simulink model "QuarterModelSimulink"  (R2017a)
settings: Solver=VariableStepAuto  StartTime=0.0  StopTime=20  RelTol=1e-3
values from neighbouring files (symbols this model uses):
  c_s = 2 * zeta * sqrt(k_u*m_s)    [simulink_main.m]
  k_s = k_u * 5    (= 34897655.371)    [simulink_main.m]
  k_u = k_u_eng * Pa_over_psi    (= 6979531.0742)    [simulink_main.m]
  m_s = 1109 / 4    (= 277.25)    [simulink_main.m]
  m_u = m_u_extra + m_rubber + m_air    [simulink_main.m]
settings Model: Creator=alexkost  LastModifiedBy=alexkost

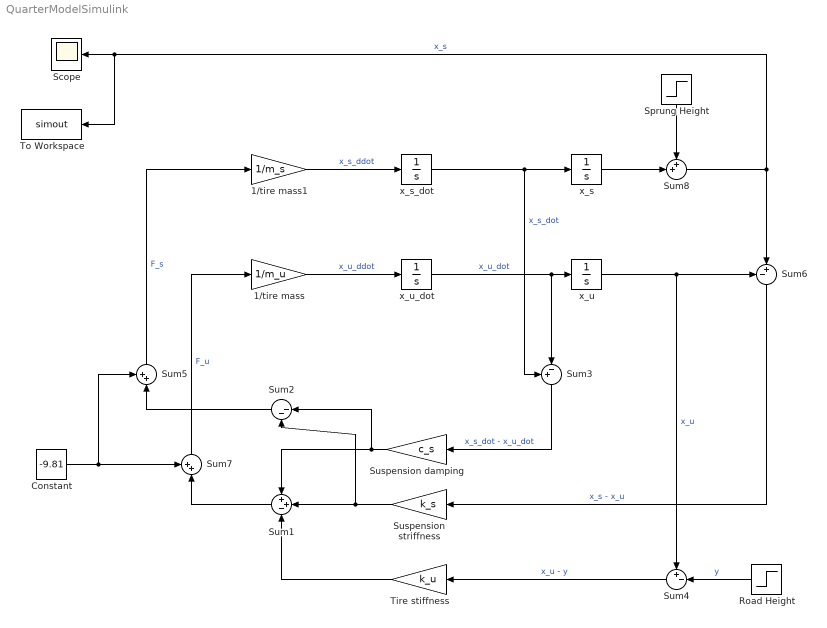
== system QuarterModelSimulink ==
  1/tire mass : Gain  Gain=1/m_u
  1/tire mass1 : Gain  Gain=1/m_s
  Constant : Constant  Value=-9.81
  Road Height : Step  After=-1  SampleTime=0
  Scope : Scope
  Sprung Height : Step  After=0  SampleTime=0
  Sum1 : Sum  Inputs=++-
  Sum2 : Sum  Inputs=|--
  Sum3 : Sum  Inputs=+-|
  Sum4 : Sum  Inputs=+-|
  Sum5 : Sum  Inputs=++|
  Sum6 : Sum  Inputs=-+|
  Sum7 : Sum  Inputs=++|
  Sum8 : Sum  Inputs=++|
  Suspension damping : Gain  Gain=c_s
  Suspension striffness : Gain  Gain=k_s
  Tire stiffness : Gain  Gain=k_u
  To Workspace : ToWorkspace  VariableName=simout  SaveFormat=Timeseries  SampleTime=-1
  x_s : Integrator
  x_s_dot : Integrator
  x_u : Integrator
  x_u_dot : Integrator
  wires:
  x_s_dot/1 -> Sum3/1, x_s/1  "x_s_dot"
  x_u_dot/1 -> Sum3/2, x_u/1  "x_u_dot"
  1/tire mass1/1 -> x_s_dot/1  "x_s_ddot"
  1/tire mass/1 -> x_u_dot/1  "x_u_ddot"
  Sum6/1 -> Suspension striffness/1  "x_s - x_u"
  x_u/1 -> Sum6/1, Sum4/1  "x_u"
  Sum3/1 -> Suspension damping/1  "x_s_dot - x_u_dot"
  Suspension damping/1 -> Sum2/1, Sum1/1
  Suspension striffness/1 -> Sum2/2, Sum1/2
  Sum4/1 -> Tire stiffness/1  "x_u - y"
  Road Height/1 -> Sum4/2  "y"
  Tire stiffness/1 -> Sum1/3
  Sum7/1 -> 1/tire mass/1  "F_u"
  Sum1/1 -> Sum7/2
  Sum2/1 -> Sum5/2
  Constant/1 -> Sum5/1, Sum7/1
  Sum5/1 -> 1/tire mass1/1  "F_s"
  x_s/1 -> Sum8/2
  Sum8/1 -> To Workspace/1, Scope/1, Sum6/2  "x_s"
  Sprung Height/1 -> Sum8/1
